simulink model "FourthCOMController"  (Simulink 7.9)
settings: Solver=ode3  StartTime=0.0  StopTime=inf  RelTol=1e-3
libraries: dspmtrx3 x5, simulink x4, simulink_extras x1, utility x1
settings Model: Creator=jorhabib  LastModifiedBy=jorhabib

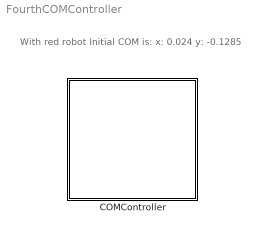
== system FourthCOMController ==
  note: With red robot Initial COM is:
      | x:  0.024
      | y:  -0.1285
  COMController : Subsystem  mask{robotName='icubSim', Ts=0.01}
      mask prompts: robotName "Robot Name"; Ts "Rate (sec)"

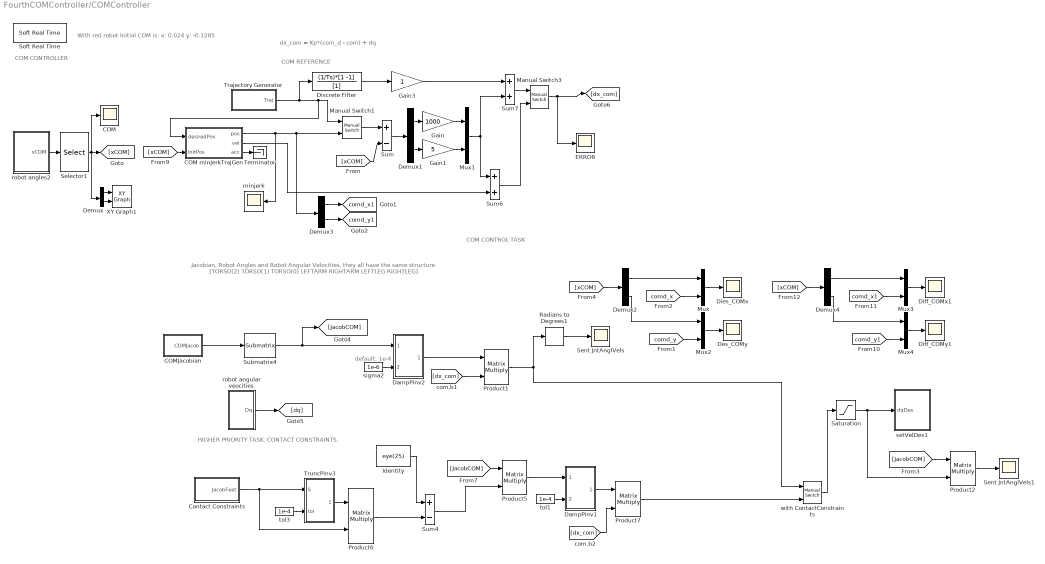
== system FourthCOMController/COMController ==
  note: COM CONTROL TASK
  note: COM CONTROLLER
  note: dx_com = Kp*(com_d - com) + dq
  note: default: 1e-4
  note: Jacobian, Robot Angles and Robot Angular Velocities, they all have the same structure
      | [TORSO(2)  TORSO(1)  TORSO(0)    LEFTARM    RIGHTARM    LEFTLEG    RIGHTLEG]
  note: COM REFERENCE
  note: HIGHER PRIORITY TASK. CONTACT CONSTRAINTS.
  note: With red robot Initial COM is:
      | x:  0.024
      | y:  -0.1285
  COM : Scope
      settings: TimeRange=100  YMin=-0.1  YMax=0.175  SaveName=ScopeData4
  COM minJerkTrajGen : Subsystem
  COMJacobian : Subsystem
  Contact Constraints : Subsystem
  DampPinv1 : Subsystem  mask{tol=1e-4}
      mask prompts: tol "Tolerance"
  DampPinv2 : Subsystem  mask{tol=1e-4}
      mask prompts: tol "Tolerance"
  Demux{,1..4} (5 alike) : Demux  Outputs=2
  Des_COMy : Scope
      settings: TimeRange=100  YMin=-0.1425  YMax=-0.1125  SaveName=ScopeData6
  Dies_COMx : Scope
      settings: TimeRange=100  YMin=0.01  YMax=0.04  SaveName=ScopeData2
  Diff_COMx1 : Scope
      settings: TimeRange=100  YMin=0.0215  YMax=0.03  SaveName=ScopeData5
  Diff_COMy1 : Scope
      settings: TimeRange=100  YMin=-0.135  YMax=-0.0925  SaveName=ScopeData7
  Discrete Filter : DiscreteFilter  Numerator=(1/Ts)*[1 -1]  Denominator=[1]
  ERROR : Scope
      settings: TimeRange=100  YMin=-0.015  YMax=0.015  SaveName=ScopeData3
  Gain : Gain  Gain=1000
  Gain1 : Gain  Gain=5
  Gain3 : Gain
  Identity : Constant  Value=eye(25)
  Manual Switch1 : simulink/Signal Routing/Manual Switch  sw=1  action=0  varsize=off
  Manual Switch3 : simulink/Signal Routing/Manual Switch  sw=1  action=0  varsize=off
  Mux{,1..4} (5 alike) : Mux  Inputs=2
  Product{1..2,5..7} (5 alike) : Product  Multiplication=Matrix(*)  RndMeth=Zero
  Radians to Degrees1 : simulink_extras/Transformations/Radians to Degrees
  Saturation : Saturate  UpperLimit=0.8  LowerLimit=-0.8
  Selector1 : Selector  IndexMode=Zero-based  InputPortWidth=7  IndexOptions=Index vector (dialog)  Indices=[0:1]  OutputSizes=1
  Sent JntAnglVels : Scope
      settings: YMin=-0.04  YMax=0.03
  Sent JntAnglVels1 : Scope
      settings: TimeRange=100  YMin=-0.01  YMax=0.01  SaveName=ScopeData8
  Soft Real Time : utility/Soft Real Time  x=Ts
  Submatrix4 : dspmtrx3/Submatrix  RowSpan=Range of rows  RowStartMode=First  RowStartIndex=1  RowEndMode=Index  RowEndIndex=2  ColSpan=Range of columns  ColStartMode=Index  ColStartIndex=7  ColEndMode=Last  ColEndIndex=6
  Sum : Sum  Inputs=+-
  Sum4 : Sum  Inputs=+-
  Sum6 : Sum
  Sum7 : Sum
  Terminator : Terminator
  Trajectory Generator : Subsystem
  TruncPinv3 : Subsystem  mask{tol=1e-4}
      mask prompts: tol "Tolerance"
  XY Graph1 : simulink/Sinks/XY Graph  xmin=0.01  xmax=0.04  ymin=-0.15  ymax=-0.115  st=-1
  minjerk : Scope
      settings: TimeRange=100  YMin=-0.12  YMax=-0.025
  robot angles2 : Subsystem
  robot angular veocities : Subsystem
  setVelDes1 : Subsystem
  sigma2 : Constant  Value=1e-6
  tol1 : Constant  Value=1e-4
  tol3 : Constant  Value=1e-4
  with ContactConstraints : simulink/Signal Routing/Manual Switch  sw=1  action=0  varsize=off
  tag scope: comd_x1=global, comd_y1=global
  wires:
  [xCOM] -> Sum/2
  Sum/1 -> Demux1/1
  Selector1/1 -> [xCOM], Demux/1, COM/1
  robot angles2/1(xCOM) -> Selector1/1
  sigma2/1 -> DampPinv2/2(sigma)
  Submatrix4/1 -> [JacobCOM], DampPinv2/1(mat)
  [dx_com] -> Product1/2
  Product1/1 -> Radians to Degrees1/1, with ContactConstraints/1
  Radians to Degrees1/1 -> Sent JntAnglVels/1
  Demux/1 -> XY Graph1/1
  Demux/2 -> XY Graph1/2
  Mux/1 -> Dies_COMx/1
  [comd_x] -> Mux/2
  Demux1/1 -> Gain/1
  Demux1/2 -> Gain1/1
  Gain/1 -> Mux1/1
  Gain1/1 -> Mux1/2
  [comd_y] -> Mux2/2
  Mux2/1 -> Des_COMy/1
  [xCOM] -> Demux2/1
  Demux2/1 -> Mux/1
  Demux2/2 -> Mux2/1
  COMJacobian/1(COMJacob) -> Submatrix4/1
  [JacobCOM] -> Product5/1
  Identity/1 -> Sum4/1
  tol3/1 -> TruncPinv3/2(tol)
  TruncPinv3/1(Tpinv) -> Product6/1
  Product6/1 -> Sum4/2
  Contact Constraints/1(JacobFeet) -> TruncPinv3/1(S), Product6/2
  Sum4/1 -> Product5/2
  Product5/1 -> DampPinv1/1(mat)
  tol1/1 -> DampPinv1/2(sigma)
  [dx_com] -> Product7/2
  Product7/1 -> with ContactConstraints/2
  with ContactConstraints/1 -> Saturation/1
  Manual Switch1/1 -> Sum/1
  Trajectory Generator/1(Traj) -> Manual Switch1/1, COM minJerkTrajGen/1(desiredPos), Discrete Filter/1
  [xCOM] -> COM minJerkTrajGen/2(initPos)
  COM minJerkTrajGen/1(pos) -> minjerk/1, Manual Switch1/2, Demux3/1
  Mux1/1 -> Sum6/1, Sum7/2
  Sum6/1 -> Manual Switch3/2
  COM minJerkTrajGen/2(vel) -> Sum6/2
  Demux3/1 -> [comd_x1]
  Demux3/2 -> [comd_y1]
  Mux3/1 -> Diff_COMx1/1
  [comd_x1] -> Mux3/2
  [comd_y1] -> Mux4/2
  Mux4/1 -> Diff_COMy1/1
  [xCOM] -> Demux4/1
  Demux4/1 -> Mux3/1
  Demux4/2 -> Mux4/1
  Discrete Filter/1 -> Gain3/1
  Sum7/1 -> Manual Switch3/1
  Manual Switch3/1 -> [dx_com], ERROR/1
  Gain3/1 -> Sum7/1
  Saturation/1 -> setVelDes1/1(dqDes), Product2/2
  [JacobCOM] -> Product2/1
  Product2/1 -> Sent JntAnglVels1/1
  DampPinv2/1(DPinv) -> Product1/1
  DampPinv1/1(DPinv) -> Product7/1
  robot angular veocities/1(Dq) -> [dq]
  COM minJerkTrajGen/3(acc) -> Terminator/1

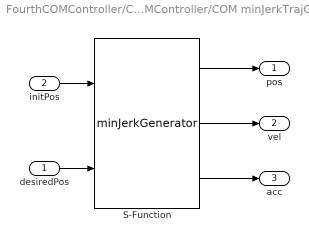
== system FourthCOMController/COMController/COM minJerkTrajGen ==
  desiredPos : Inport
  initPos : Inport  Port=2
  S-Function : S-Function  FunctionName=minJerkGenerator  Parameters=dim, rate, tt  EnableBusSupport=off  mask{dim=2, rate=10, tt=30}
      mask prompts: dim "Trajectory dimension (int)"; rate "Simulation rate (int) [ms]"; tt "Trajectory time [s]"
  pos : Outport
  vel : Outport  Port=2
  acc : Outport  Port=3
  wires:
  desiredPos/1 -> S-Function/2
  initPos/1 -> S-Function/1
  S-Function/3 -> acc/1
  S-Function/1 -> pos/1
  S-Function/2 -> vel/1

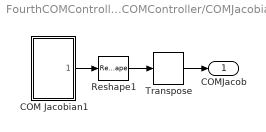
== system FourthCOMController/COMController/COMJacobian ==
  COM Jacobian1 : Subsystem
  Reshape1 : Reshape  OutputDimensionality=Customize  OutputDimensions=[31,6]
  Transpose : dspmtrx3/Transpose  Hermitian=off  overflowFlag=off
  COMJacob : Outport
  wires:
  COM Jacobian1/1(Jacobian) -> Reshape1/1
  Reshape1/1 -> Transpose/1
  Transpose/1 -> COMJacob/1

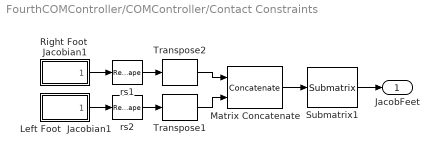
== system FourthCOMController/COMController/Contact Constraints ==
  Left Foot  Jacobian1 : Subsystem
  Matrix Concatenate : Concatenate  Mode=Multidimensional array
  Right Foot  Jacobian1 : Subsystem
  Submatrix1 : dspmtrx3/Submatrix  RowSpan=Range of rows  RowStartMode=First  RowStartIndex=1  RowEndMode=Index  RowEndIndex=2  ColSpan=Range of columns  ColStartMode=Index  ColStartIndex=7  ColEndMode=Last  ColEndIndex=6
  Transpose1 : dspmtrx3/Transpose  Hermitian=off  overflowFlag=off
  Transpose2 : dspmtrx3/Transpose  Hermitian=off  overflowFlag=off
  rs1 : Reshape  OutputDimensionality=Customize  OutputDimensions=[31,6]
  rs2 : Reshape  OutputDimensionality=Customize  OutputDimensions=[31,6]
  JacobFeet : Outport
  wires:
  Right Foot  Jacobian1/1(Jacobian) -> rs1/1
  Left Foot  Jacobian1/1(Jacobian) -> rs2/1
  rs1/1 -> Transpose2/1
  rs2/1 -> Transpose1/1
  Transpose2/1 -> Matrix Concatenate/1
  Transpose1/1 -> Matrix Concatenate/2
  Matrix Concatenate/1 -> Submatrix1/1
  Submatrix1/1 -> JacobFeet/1

== system FourthCOMController/COMController/DampPinv1 ==
  mat : Inport
  sigma : Inport  Port=2
  Damped Pseudo Inverse : MATLAB Function  TreatAsAtomicUnit=on
  DPinv : Outport
  wires:
  mat/1 -> Damped Pseudo Inverse/1(mat)
  Damped Pseudo Inverse/1(DPinv) -> DPinv/1
  sigma/1 -> Damped Pseudo Inverse/2(sigma)

== system FourthCOMController/COMController/DampPinv2 ==
  mat : Inport
  sigma : Inport  Port=2
  Damped Pseudo Inverse : MATLAB Function  TreatAsAtomicUnit=on
  DPinv : Outport
  wires:
  sigma/1 -> Damped Pseudo Inverse/2(sigma)
  Damped Pseudo Inverse/1(DPinv) -> DPinv/1
  mat/1 -> Damped Pseudo Inverse/1(mat)

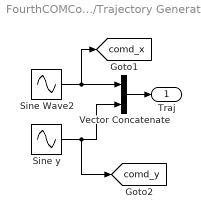
== system FourthCOMController/COMController/Trajectory Generator ==
  Sine Wave2 : Sin  Amplitude=0.01  Bias=0.02407  Frequency=0.2  Phase=pi/2
  Sine y : Sin  Amplitude=0.01  Bias=-0.1287  Frequency=0.2
  Vector Concatenate : Concatenate
  Traj : Outport
  tag scope: comd_x=global, comd_y=global
  wires:
  Sine Wave2/1 -> Vector Concatenate/1, [comd_x]
  Sine y/1 -> Vector Concatenate/2, [comd_y]
  Vector Concatenate/1 -> Traj/1

== system FourthCOMController/COMController/TruncPinv3 ==
  S : Inport
  tol : Inport  Port=2
  Truncated PseudoInverse : MATLAB Function  TreatAsAtomicUnit=on
  Tpinv : Outport
  wires:
  tol/1 -> Truncated PseudoInverse/2(tol)
  Truncated PseudoInverse/1(TPinv) -> Tpinv/1
  S/1 -> Truncated PseudoInverse/1(mat)

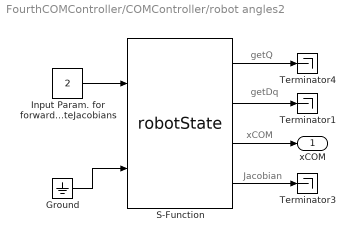
== system FourthCOMController/COMController/robot angles2 ==
  note: getDq
  note: xCOM
  note: getQ
  note: Jacobian
  Ground : Ground
  "Input Param. for forwardKinematics and  computeJacobians " : Constant  Value=2  OutDataTypeStr=int8
  S-Function : S-Function  FunctionName=robotState  Parameters=val,robotname,localname  EnableBusSupport=off  mask{val=2, robotname=robotName, localname='robotState'}
      mask prompts: val "Value"; robotname "Robot Name (icub - icubSim)"; localname "Module Name"
  Terminator1 : Terminator
  Terminator3 : Terminator
  Terminator4 : Terminator
  xCOM : Outport
  wires:
  Ground/1 -> S-Function/2
  S-Function/2 -> Terminator1/1
  S-Function/1 -> Terminator4/1
  S-Function/3 -> xCOM/1
  "Input Param. for forwardKinematics and  computeJacobians "/1 -> S-Function/1
  S-Function/4 -> Terminator3/1

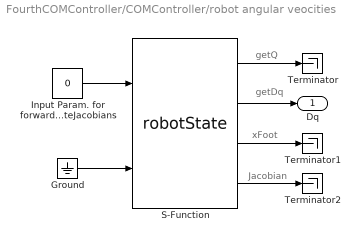
== system FourthCOMController/COMController/robot angular veocities ==
  note: Jacobian
  note: getQ
  note: xFoot
  note: getDq
  Ground : Ground
  "Input Param. for forwardKinematics and  computeJacobians " : Constant  Value=0  OutDataTypeStr=int8
  S-Function : S-Function  FunctionName=robotState  Parameters=val,robotname,localname  EnableBusSupport=off  mask{val=1, robotname='icubSim', localname='robotState'}
      mask prompts: val "Value"; robotname "Robot Name (icub - icubSim)"; localname "Module Name"
  Terminator : Terminator
  Terminator1 : Terminator
  Terminator2 : Terminator
  Dq : Outport
  wires:
  S-Function/4 -> Terminator2/1
  "Input Param. for forwardKinematics and  computeJacobians "/1 -> S-Function/1
  S-Function/3 -> Terminator1/1
  S-Function/1 -> Terminator/1
  S-Function/2 -> Dq/1
  Ground/1 -> S-Function/2

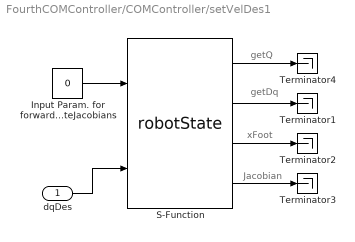
== system FourthCOMController/COMController/setVelDes1 ==
  note: getDq
  note: xFoot
  note: getQ
  note: Jacobian
  dqDes : Inport
  "Input Param. for forwardKinematics and  computeJacobians " : Constant  Value=0  OutDataTypeStr=int8
  S-Function : S-Function  FunctionName=robotState  Parameters=val,robotname,localname  EnableBusSupport=off  mask{val=4, robotname=robotName, localname='robotState'}
      mask prompts: val "Value"; robotname "Robot Name (icub - icubSim)"; localname "Module Name"
  Terminator{1..4} (4 alike) : Terminator
  wires:
  dqDes/1 -> S-Function/2
  S-Function/2 -> Terminator1/1
  S-Function/1 -> Terminator4/1
  S-Function/3 -> Terminator2/1
  "Input Param. for forwardKinematics and  computeJacobians "/1 -> S-Function/1
  S-Function/4 -> Terminator3/1

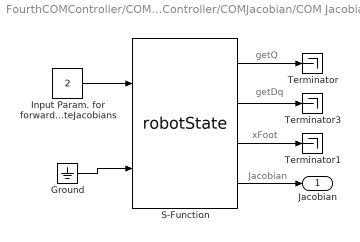
== system FourthCOMController/COMController/COMJacobian/COM Jacobian1 ==
  note: getDq
  note: xFoot
  note: getQ
  note: Jacobian
  Ground : Ground
  "Input Param. for forwardKinematics and  computeJacobians " : Constant  Value=2  OutDataTypeStr=int8
  S-Function : S-Function  FunctionName=robotState  Parameters=val,robotname,localname  EnableBusSupport=off  mask{val=3, robotname=robotName, localname='robotState'}
      mask prompts: val "Value"; robotname "Robot Name (icub - icubSim)"; localname "Module Name"
  Terminator : Terminator
  Terminator1 : Terminator
  Terminator3 : Terminator
  Jacobian : Outport
  wires:
  Ground/1 -> S-Function/2
  S-Function/2 -> Terminator3/1
  S-Function/1 -> Terminator/1
  S-Function/3 -> Terminator1/1
  "Input Param. for forwardKinematics and  computeJacobians "/1 -> S-Function/1
  S-Function/4 -> Jacobian/1

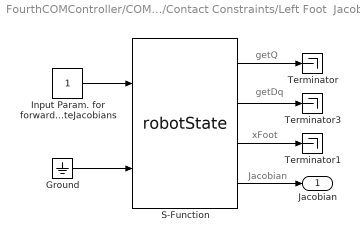
== system FourthCOMController/COMController/Contact Constraints/Left Foot  Jacobian1 ==
  note: Jacobian
  note: getQ
  note: xFoot
  note: getDq
  Ground : Ground
  "Input Param. for forwardKinematics and  computeJacobians " : Constant  OutDataTypeStr=int8
  S-Function : S-Function  FunctionName=robotState  Parameters=val,robotname,localname  EnableBusSupport=off  mask{val=3, robotname=robotName, localname='robotState'}
      mask prompts: val "Value"; robotname "Robot Name (icub - icubSim)"; localname "Module Name"
  Terminator : Terminator
  Terminator1 : Terminator
  Terminator3 : Terminator
  Jacobian : Outport
  wires:
  S-Function/4 -> Jacobian/1
  "Input Param. for forwardKinematics and  computeJacobians "/1 -> S-Function/1
  S-Function/3 -> Terminator1/1
  S-Function/1 -> Terminator/1
  S-Function/2 -> Terminator3/1
  Ground/1 -> S-Function/2

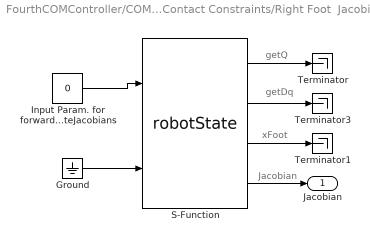
== system FourthCOMController/COMController/Contact Constraints/Right Foot  Jacobian1 ==
  note: getDq
  note: xFoot
  note: getQ
  note: Jacobian
  Ground : Ground
  "Input Param. for forwardKinematics and  computeJacobians " : Constant  Value=0  OutDataTypeStr=int8
  S-Function : S-Function  FunctionName=robotState  Parameters=val,robotname,localname  EnableBusSupport=off  mask{val=3, robotname=robotName, localname='robotState'}
      mask prompts: val "Value"; robotname "Robot Name (icub - icubSim)"; localname "Module Name"
  Terminator : Terminator
  Terminator1 : Terminator
  Terminator3 : Terminator
  Jacobian : Outport
  wires:
  S-Function/2 -> Terminator3/1
  S-Function/1 -> Terminator/1
  S-Function/3 -> Terminator1/1
  "Input Param. for forwardKinematics and  computeJacobians "/1 -> S-Function/1
  S-Function/4 -> Jacobian/1
  Ground/1 -> S-Function/2

== matlab function COMController/DampPinv2/Damped Pseudo Inverse ==
  data: mat input double; DPinv output double; sigma input double
function DPinv  = fcn(mat,sigma)
% % Economy size svd of mat
% [U,S,V] = svd(mat,'econ');
% % Damped version of S with sigma
% S(S>sigma)=S(S>sigma)./((S(S>sigma)).^2+sigma^2);
% % Damped pseudoinverse
% DPinv = V*pinv(S)*U';

% Economy size svd of mat
[U,S,V] = svd(mat,'econ');
% Damped version of S with sigma
S(logical(eye(length(S))))=S(logical(eye(length(S))))./((S(logical(eye(length(S))))).^2+sigma^2);
% Damped pseudoinverse
DPinv = V*pinv(S)*U';

== matlab function COMController/DampPinv1/Damped Pseudo Inverse ==
  data: mat input double; DPinv output double; sigma input double
function DPinv  = fcn(mat,sigma)
% Economy size svd of mat
[U,S,V] = svd(mat,'econ');
% Damped version of S with sigma
S(S>sigma)=S(S>sigma)./((S(S>sigma)).^2+sigma^2);
% Damped pseudoinverse
DPinv = V*pinv(S)*U';

== matlab function COMController/TruncPinv3/Truncated PseudoInverse ==
  data: mat input double; TPinv output double; tol input double
function TPinv  = fcn(mat,tol)
%#codegen
[U,S,V] = svd(mat,'econ');
% Setting to 1/S(i,i) singular values greater than tol
 S(S>tol)=1./S(S>tol);
TPinv = V*pinv(S)*U';
